simulink model "block_diagram_PMDC"  (R2023b)
settings: Solver=VariableStepAuto  StartTime=0.0  StopTime=0.5  RelTol=1e-3
values from neighbouring files (symbols this model uses):
  Bm = 0.00000604    (= 6.04e-06)    [setup_params_pmdc.m]
  J = 0.00000161    (= 1.61e-06)    [setup_params_pmdc.m]
  Kv = 0.0141    [setup_params_pmdc.m]
  LAA = 0.12    [setup_params_pmdc.m]
  ra = 7    [setup_params_pmdc.m]
  Tl = 0.003    [setup_params_pmdc.m]
  Va = 6    [setup_params_pmdc.m]
settings Model: Creator=Noor  LastModifiedBy=USER
settings SolverCC: AlgebraicLoopSolver=TrustRegion
settings DataIOCC: ReturnWorkspaceOutputs=off
settings DebuggingCC: UnconnectedInputMsg=warning  UnconnectedOutputMsg=warning  UnconnectedLineMsg=warning  ArithmeticOperatorsInVariantConditions=warning
settings ModelReferenceCC: EnableRefExpFcnMdlSchedulingChecks=on
settings SFSimCC: SimUseLocalCustomCode=off  CustomCodeUndefinedFunction=UseInterfaceOnly
settings RTWCC: RTWUseLocalCustomCode=off

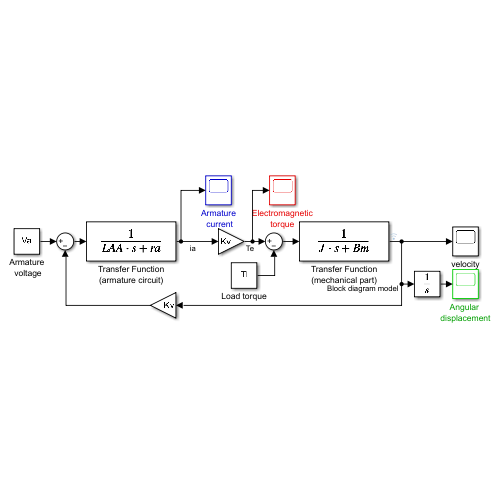
[thumbnail: Simulink's stored preview of the top-level diagram]
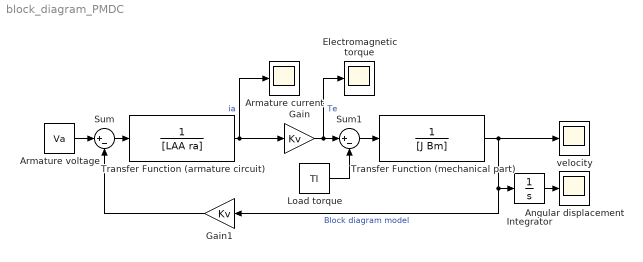
== system block_diagram_PMDC ==
  Angular displacement : Scope
  Armature current : Scope
  Armature voltage : Constant  Value=Va
  "Electromagnetic torque " : Scope
  Gain : Gain  Gain=Kv
  Gain1 : Gain  Gain=Kv
  Integrator : Integrator
  Load torque : Constant  Value=Tl
  Sum : Sum  Inputs=|+-
  Sum1 : Sum  Inputs=|+-
  Transfer Function (armature circuit) : TransferFcn  Denominator=[LAA ra]
  Transfer Function (mechanical part) : TransferFcn  Denominator=[J Bm]
  velocity : Scope
  wires:
  Gain/1 -> Sum1/1, "Electromagnetic torque "/1  "Te"
  Transfer Function (armature circuit)/1 -> Gain/1, Armature current/1  "ia"
  Sum/1 -> Transfer Function (armature circuit)/1
  Sum1/1 -> Transfer Function (mechanical part)/1
  Transfer Function (mechanical part)/1 -> velocity/1, Integrator/1, Gain1/1  "Block diagram model"
  Gain1/1 -> Sum/2
  Armature voltage/1 -> Sum/1
  Integrator/1 -> Angular displacement/1
  Load torque/1 -> Sum1/2
